simulink model "kinovaMicoSimscapeModel"  (R2021b)
settings: Solver=VariableStepAuto  StartTime=0.0  StopTime=0.3  FixedStep=0.01  RelTol=1e-3
PostLoadFcn:
  | micoRigidBodyTreeCreation;
  | IC=deg2rad([-90,180,180,0,0,0]);
  | interactiveHomePosition=deg2rad([-90 90 177.5 90 0 0]');
  | load("./KinovaMicoSimscapeVariantConfigurations.mat");
values from neighbouring files (symbols this model uses):
  micoCandlePosition = deg2rad([0,180,180,0,0,0])    [KinovaMicoSimscapeInitializeScript.m]    (also in generatingRandomTrajectory.m)
  ViaPointsTaskSpace = [ViaPointsTaskSpace;[[pi;0;pi],[pi;0;pi],[pi;0;pi],[pi;0;pi],[0;0;0],[0;0;0],[pi;0;pi]]]    [KinovaMicoSimscapeInitializeScript.m]    (also in generatingRandomTrajectory.m = [ViaPointsTaskSpace;zeros(3,7)])
undefined symbols (not defined in the file or in its folder): Mico, ViaPointsJointSpace, X, Y, Z
libraries: sm_lib x26, nesl_utility x19, robotcorelib x4, robotmaniplib x3, pid_lib x2
(part 23 of 50)

== matlab function kinovaMicoSimscapeModel/Variant Subsystem/JointSpaceController/Sliding Adaptive Control/VectorManipulation ==
  data: S output; q input; dqr output; dq input; qd input; dqd input; ddqd input; ddqr output
function [S,dqr,ddqr] = VectorManipulation(q,dq,qd,dqd,ddqd)
%% Unpacking the measurements/desired points
qError=q-qd;
dqError=dq-dqd;

%Define parameters
lambda=1*eye(6);

dqr=dqd-lambda*qError;
ddqr=ddqd-lambda*dqError;

%Define sliding surface
S=dqError+lambda*qError;
